simulink model "fahrenheitConverter_Rafael_Enriquez"  (R2022b)
settings: Solver=VariableStepAuto  StartTime=0.0  StopTime=10.0  RelTol=1e-3
settings Model: Creator=fitir  LastModifiedBy=fitir

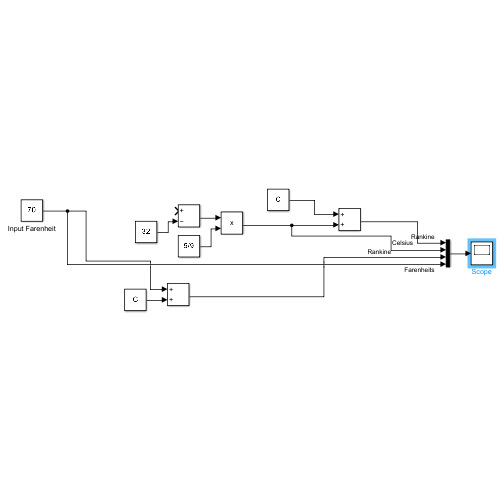
[thumbnail: Simulink's stored preview of the top-level diagram]
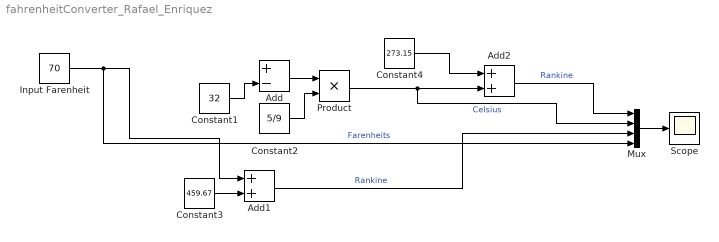
== system fahrenheitConverter_Rafael_Enriquez ==
  Add : Sum  Inputs=+-
  Add1 : Sum
  Add2 : Sum
  Constant1 : Constant  Value=32  SampleTime=1
  Constant2 : Constant  Value=5/9  SampleTime=1
  Constant3 : Constant  Value=459.67  SampleTime=1
  Constant4 : Constant  Value=273.15  SampleTime=1
  Input Farenheit : Constant  Value=70  SampleTime=1
  Mux : Mux
  Product : Product
  Scope : Scope
  wires:
  Input Farenheit/1 -> Mux/4, Add1/1  "Farenheits"
  Constant1/1 -> Add/2
  Add/1 -> Product/1
  Constant2/1 -> Product/2
  Constant3/1 -> Add1/2
  Constant4/1 -> Add2/1
  Add2/1 -> Mux/1  "Rankine"
  Product/1 -> Add2/2, Mux/2  "Celsius"
  Add1/1 -> Mux/3  "Rankine"
  Mux/1 -> Scope/1
